simulink model "ClosedLoop_ssPlant_Kcont"  (R2018b)
settings: Solver=ode4  StartTime=0.0  StopTime=10  FixedStep=0.005  RelTol=1e-3
settings Model: Creator=manzand  LastModifiedBy=manzand
settings SFSimCC: SimUseLocalCustomCode=off
settings RTWCC: RTWUseLocalCustomCode=off
settings CodeAppCC: StateflowObjectComments=on

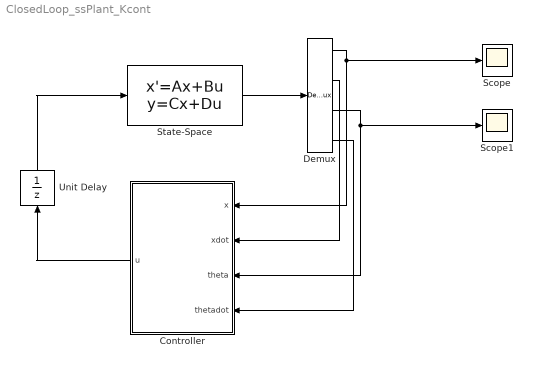
== system ClosedLoop_ssPlant_Kcont ==
  Controller : Subsystem
  Demux : Demux
  Scope : Scope
  Scope1 : Scope
  State-Space : StateSpace  A=|  B=|  C=|  D=|  InitialCondition=[1000 1000 1000 1000]
      A=|
      | [-70.9075641724949	-142.716008423025	-127.437066945202	248.294128957997;
      | -3.03592637405808	-10.3288709732968	-0.493815798669647	21.1354434753889;
      | 0.670981876929746	-7.23294283690567	-2.47413975251526	9.96796971175632;
      | 0.200385870404734	1.55316407844718	0.370840249908544	-3.66739535937049]
      B=|
      | [-0.0348457430523765;
      | -0.630599300367353;
      | -0.124983752737534;
      | -0.507159367596411]
      C=|
      | [-2.06371202902639e-06	0.000285173392916046	0.000369531172924105	0.00263539784891988;
      | 2.82106671085145e-05	-0.000612768936893908	9.30825895865964e-05	-0.000231543767866056;
      | -6.54522748496599e-07	-1.26245836377179e-06	-0.000128108505970310	-6.25961435597254e-05;
      | -2.41399172816718e-05	0.000467823843620001	0.000188796774982193	-0.000618392394704504]
      D=|
      | [3.90004839716945e-06;
      | -1.23902360268618e-06;
      | -1.21326595221446e-07;
      | 2.27036604040985e-08]
  Unit Delay : UnitDelay  SampleTime=0.005
  wires:
  State-Space/1 -> Demux/1
  Demux/1 -> Scope/1, Controller/1(x)
  Demux/2 -> Controller/2(xdot)
  Demux/3 -> Scope1/1, Controller/3(theta)
  Demux/4 -> Controller/4(thetadot)
  Controller/1(u) -> Unit Delay/1
  Unit Delay/1 -> State-Space/1

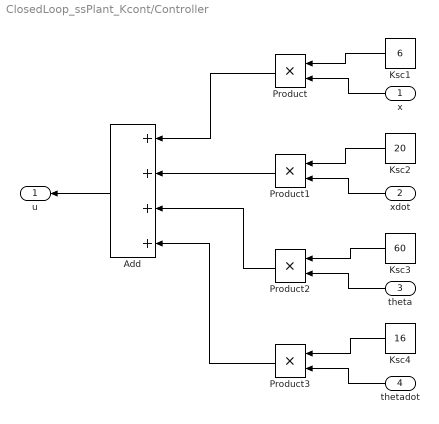
== system ClosedLoop_ssPlant_Kcont/Controller ==
  x : Inport
  xdot : Inport  Port=2
  theta : Inport  Port=3
  thetadot : Inport  Port=4
  Add : Sum  Inputs=++++
  Ksc1 : Constant  Value=6
  Ksc2 : Constant  Value=20
  Ksc3 : Constant  Value=60
  Ksc4 : Constant  Value=16
  Product{,1..3} (4 alike) : Product
  u : Outport
  wires:
  theta/1 -> Product2/2
  Ksc4/1 -> Product3/1
  Ksc1/1 -> Product/1
  xdot/1 -> Product1/2
  Ksc2/1 -> Product1/1
  x/1 -> Product/2
  thetadot/1 -> Product3/2
  Ksc3/1 -> Product2/1
  Product/1 -> Add/1
  Product3/1 -> Add/4
  Product2/1 -> Add/3
  Add/1 -> u/1
  Product1/1 -> Add/2
